simulink model "P7_son2"  (R2021b)
settings: Solver=VariableStepAuto  StartTime=0.0  StopTime=10.0  RelTol=1e-3
undefined symbols (not defined in the file or in its folder): k11, k12, k21, k22, k31, k32, k41, k42, k43, sample_time
libraries: simulink x1
settings Model: Creator=11639  LastModifiedBy=11639

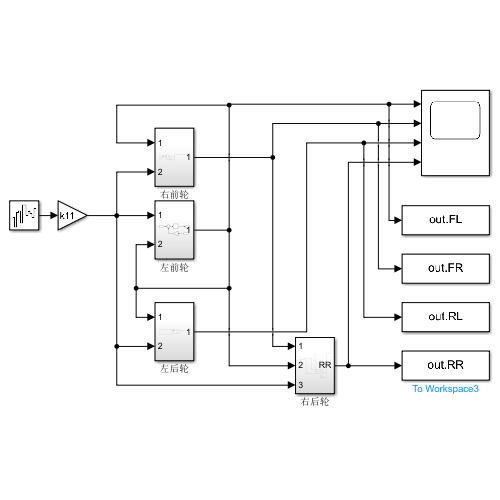
[thumbnail: Simulink's stored preview of the top-level diagram]
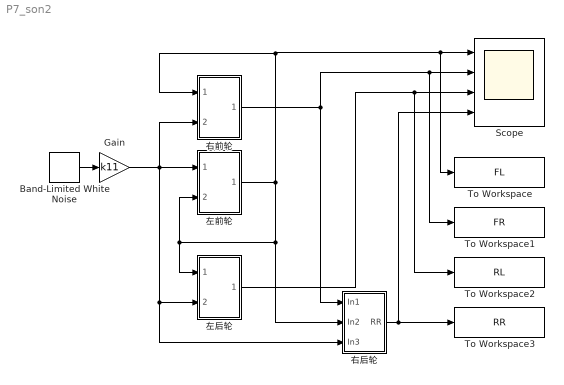
== system P7_son2 ==
  Band-Limited White Noise : simulink/Sources/Band-Limited White Noise  Cov=noise_power  Ts=sample_time  seed=seed
  Gain : Gain  Gain=k11
  Scope : Scope  NumInputPorts=4
  To Workspace : ToWorkspace  VariableName=FL  SaveFormat=Timeseries  SampleTime=-1
  To Workspace1 : ToWorkspace  VariableName=FR  SaveFormat=Timeseries  SampleTime=-1
  To Workspace2 : ToWorkspace  VariableName=RL  SaveFormat=Timeseries  SampleTime=-1
  To Workspace3 : ToWorkspace  VariableName=RR  SaveFormat=Timeseries  SampleTime=-1
  右前轮 : Subsystem
  右后轮 : Subsystem
  左前轮 : Subsystem
  左后轮 : Subsystem
  wires:
  Band-Limited White Noise/1 -> Gain/1
  Gain/1 -> 右后轮/3(In3), 左后轮/2(In2), 左前轮/1(In1), 右前轮/2(In2)
  左后轮/1(Out1) -> To Workspace2/1, Scope/3
  右前轮/1(Out1) -> 右后轮/1(In1), To Workspace1/1, Scope/2
  右后轮/1(RR) -> To Workspace3/1, Scope/4
  左前轮/1(Out1) -> 左后轮/1(In1), 左前轮/2(In2), 右后轮/2(In2), 右前轮/1(In1), To Workspace/1, Scope/1

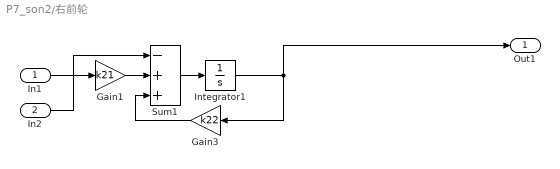
== system P7_son2/右前轮 ==
  In1 : Inport
  In2 : Inport  Port=2
  Gain1 : Gain  Gain=k21
  Gain3 : Gain  Gain=k22
  Integrator1 : Integrator
  Sum1 : Sum  Inputs=-++
  Out1 : Outport
  wires:
  Gain3/1 -> Sum1/3
  Integrator1/1 -> Out1/1, Gain3/1
  In2/1 -> Sum1/1
  Sum1/1 -> Integrator1/1
  In1/1 -> Gain1/1
  Gain1/1 -> Sum1/2

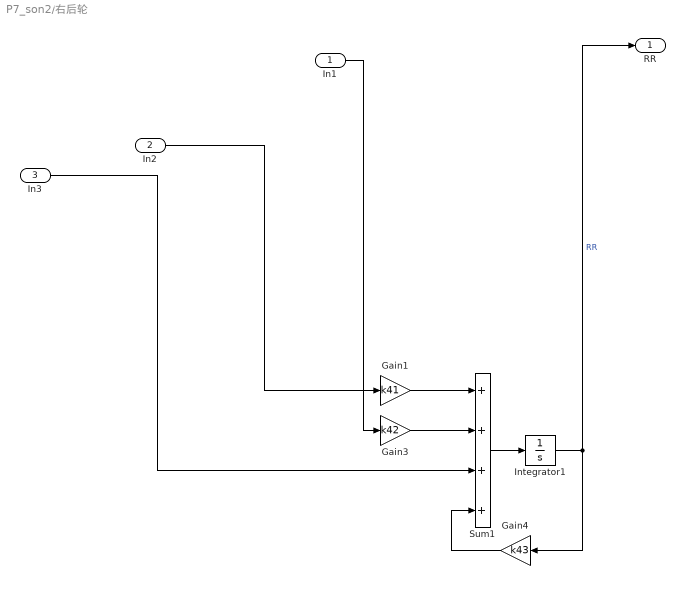
== system P7_son2/右后轮 ==
  In1 : Inport
  In2 : Inport  Port=2
  In3 : Inport  Port=3
  Gain1 : Gain  Gain=k41
  Gain3 : Gain  Gain=k42
  Gain4 : Gain  Gain=k43
  Integrator1 : Integrator
  Sum1 : Sum  Inputs=++++
  RR : Outport
  wires:
  Gain1/1 -> Sum1/1
  In1/1 -> Gain3/1
  Gain3/1 -> Sum1/2
  Integrator1/1 -> RR/1, Gain4/1  "RR"
  In2/1 -> Gain1/1
  In3/1 -> Sum1/3
  Gain4/1 -> Sum1/4
  Sum1/1 -> Integrator1/1

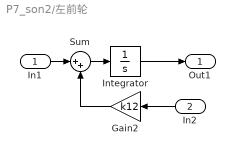
== system P7_son2/左前轮 ==
  In1 : Inport
  In2 : Inport  Port=2
  Gain2 : Gain  Gain=k12
  Integrator : Integrator
  Sum : Sum  Inputs=|++
  Out1 : Outport
  wires:
  Sum/1 -> Integrator/1
  In2/1 -> Gain2/1
  In1/1 -> Sum/1
  Gain2/1 -> Sum/2
  Integrator/1 -> Out1/1

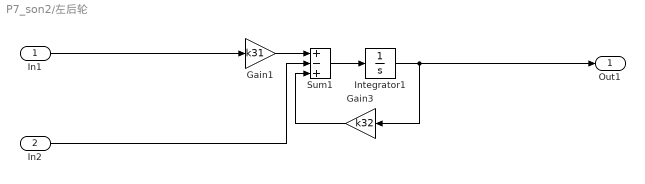
== system P7_son2/左后轮 ==
  In1 : Inport
  In2 : Inport  Port=2
  Gain1 : Gain  Gain=k31
  Gain3 : Gain  Gain=k32
  Integrator1 : Integrator
  Sum1 : Sum  Inputs=+-+
  Out1 : Outport
  wires:
  Gain3/1 -> Sum1/3
  In2/1 -> Sum1/2
  Integrator1/1 -> Out1/1, Gain3/1
  In1/1 -> Gain1/1
  Sum1/1 -> Integrator1/1
  Gain1/1 -> Sum1/1
